simulink model "H2DFRL_LExCI_env_TD3_nosfb"  (R2023a)
settings: Solver=FixedStepAuto  StartTime=0.0  StopTime=50  FixedStep=0.08  RelTol=1e-3
values from neighbouring files (symbols this model uses):
  action_mean_selector_ppo = 1:num_actions    [ReinforcementLearningBlockInit_H2DFRL.m]
  action_sampling_mode = 1    [ReinforcementLearningBlockInit_H2DFRL.m]
  action_selector_ddpg = 1:num_actions    [ReinforcementLearningBlockInit_H2DFRL.m]
  action_std_selector_ppo = 1:num_actions    [ReinforcementLearningBlockInit_H2DFRL.m]
  action_type = 1    [ReinforcementLearningBlockInit_H2DFRL.m]
  C2C_NMPC = init_C2C_NMPC_H2DF(C2C_NMPC.expdata)    [init_H2DFRL_GRU.m]
  LowerLimit = ([0.17e-3;350;-1;1.5e-3] - C2C_NMPC.Normalization.controls.mean)./(C2C_NMPC.Normalization.controls.std)    [init_H2DFRL_GRU.m]
  num_actions = 4    [ReinforcementLearningBlockInit_H2DFRL.m]
  rl_algorithm = 2    [ReinforcementLearningBlockInit_H2DFRL.m]
  Ts = 0.08    [init_H2DFRL_GRU.m]
  UpperLimit = ([0.5e-3;900;0;5.5e-3] - C2C_NMPC.Normalization.controls.mean)./(C2C_NMPC.Normalization.controls.std)    [init_H2DFRL_GRU.m]
undefined symbols (not defined in the file or in its folder): CA50_offset, DiscIntNeverNeededParam, enable_CA50_noise, enable_CA50_offset, enable_IMEP_noise, enable_IMEP_offset, IMEP_offset, NUMBER_OF_ACTIONS
libraries: simulink x15, dspsrcs4 x4, slctrlblks x2, statsLibrary x1
(part 2 of 4)

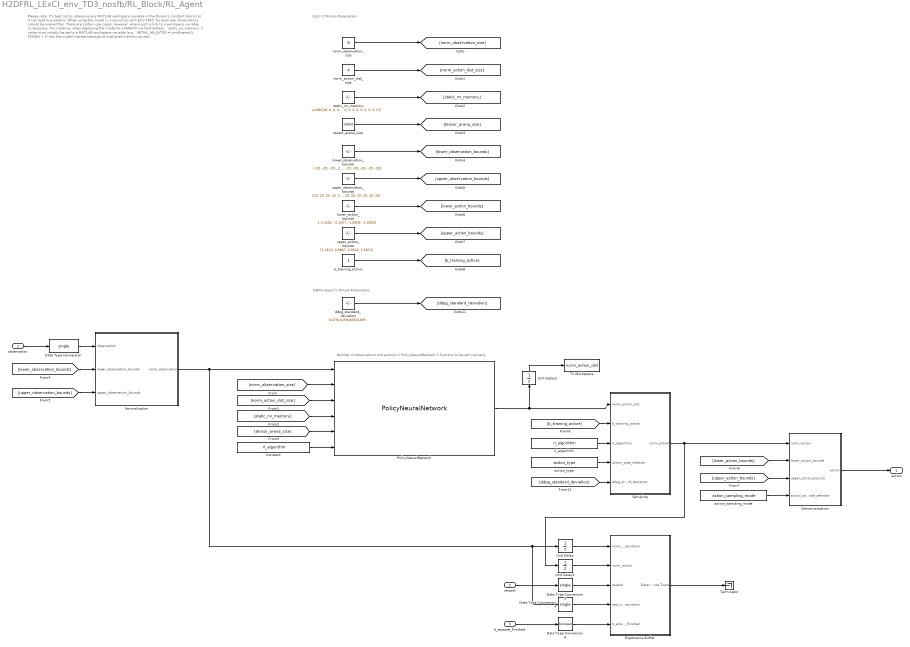
== system H2DFRL_LExCI_env_TD3_nosfb/RL_Block/RL_Agent ==
  note: LExCI 2 Minion Parameters
  note: DDPG-Specific Minion Parameters
  note: Number of observations and actions in PolicyNeuralNetwork S-Function to be set manually.
  note: Please note:
      |
      | It's best not to reference any MATLAB workspace variable in the Minion's constant blocks as it can lead to
      | problems. When using the model in conjunction with ECU-TEST, for example, those blocks cannot be
      | overwritten.
      |
      | There are certain use-cases, however, where such a link to a workspace variable is necessary. For
      | instance, when deploying the model to a MABXIII via ControlDesk, `static_nn_memory`'s value must
      | initially be set to a MATLAB workspace variable (e.g. `INITIAL_NN_BYTES = uint8(zeros(1, 65536))`). If
      | not, the model crashes because of unaligned memory access.
  observation : Inport
  reward : Inport  Port=2
  b_episode_finished : Inport  Port=3
  Constant : Constant  Value=rl_algorithm  OutDataTypeStr=uint32
  Data Type Conversion : DataTypeConversion  OutDataTypeStr=single  SaturateOnIntegerOverflow=off  RndMeth=Floor
  Data Type Conversion3 : DataTypeConversion  OutDataTypeStr=single  SaturateOnIntegerOverflow=off  RndMeth=Floor
  Data Type Conversion4 : DataTypeConversion  OutDataTypeStr=single  SaturateOnIntegerOverflow=off  RndMeth=Floor
  Data Type Conversion6 : DataTypeConversion  OutDataTypeStr=boolean  SaturateOnIntegerOverflow=off  RndMeth=Floor
  Denormalization : Subsystem
  Experience Buffer : Subsystem
  Normalization : Subsystem
  PolicyNeuralNetwork : S-Function  InitFcn=try, set_param(gcb,'FunctionName','PolicyNeuralNetwork'), end  FunctionName=PolicyNeuralNetwork  SFunctionModules=PolicyNeuralNetwork_wrapper.cpp activations activations_common add add_common add_n arg_min_max assign_variable batch_to_space_nd broadcast_args broadcast_to call_once cast ceil circular_buffer circular_buffer_common comparisons concatenation conv conv_common cumsum depth_to_space depthwise_conv depthwise_conv_common dequantize dequantize_common detection_postprocess div elementwise elu ethosu exp expand_dims fill floor floor_div floor_mod fully_connected fully_connected_common gather gather_nd hard_swish hard_swish_common if kernel_runner kernel_util_micro l2norm l2_pool_2d leaky_relu leaky_relu_common logical logical_common logistic logistic_common log_softmax lstm_eval maximum_minimum micro_tensor_utils mirror_pad mul mul_common neg pack pad pooling pooling_common prelu prelu_common quantize quantize_common read_variable reduce reduce_common reshape resize_bilinear resize_nearest_neighbor round shape slice softmax softmax_common space_to_batch_nd space_to_depth split split_v squared_difference squeeze strided_slice sub sub_common svdf svdf_common tanh transpose transpose_conv unidirectional_sequence_lstm unpack var_handle while zeros_like flatbuffer_conversions op_resolver tensor_utils error_reporter schema_utils kernel_util portable_tensor_utils quantization_util common memory_helpers all_ops_resolver micro_graph micro_error_reporter micro_context micro_profiler test_helpers recording_micro_allocator micro_interpreter micro_time micro_resource_variable test_helper_custom_ops flatbuffer_utils mock_micro_graph debug_log micro_allocation_info system_setup micro_allocator micro_string micro_utils fake_micro_context persistent_arena_buffer_allocator recording_single_arena_buffer_allocator non_persistent_arena_buffer_allocator single_arena_buffer_allocator greedy_memory_planner linear_memory_planner non_persistent_buffer_planner_shim  SFunctionDeploymentMode=off  EnableBusSupport=off  mask(S-Function Builder){}
      mask help: Simulink:masks:SFunctionBuilder_MD
      mask init:
      | val = [[.9  0.75 0.75 1 1 .9 .9 1]',[1 1 0.75 0.75 .9 .9 1 .9]'];try , sys = get_param(gcb,'SfunBuilderFcnName');if isempty(sys), sys = get_param(gcb,'FunctionName'); end,catch, sys = get_param(gcb,'FunctionName'); end
      settings: CopyFcn=set_param(gcbh,'LinkStatus','none')  PreSaveFcn=try, set_param(gcb,'FunctionName','PolicyNeuralNetwork'), end  OpenFcn=sfunctionwizard(gcbh)
      mask Display: plot(val(:,1),val(:,2)),disp(sys),port_label('input',1,'norm_observation'),port_label('input',2,'norm_observation_size'),port_label('input',3,'norm_action_dist_size'),port_label('input',4,'static_nn_memory'),port_label('input',5,'tensor_arena_size'),port_label('input',6,'rl_algorithm'),port_label('output',1,'norm_action_dist')
  Sampling : Subsystem
  Terminator : Terminator
  To Workspace : ToWorkspace  VariableName=norm_action_dist  SampleTime=-1
  Unit Delay : UnitDelay  InitialCondition=-1*ones(8,1)  SampleTime=-1  HasFrameUpgradeWarning=on
  Unit Delay1 : UnitDelay  InitialCondition=-1*ones(4,1)  SampleTime=-1  HasFrameUpgradeWarning=on
  Unit Delay2 : UnitDelay  InitialCondition=-1*ones(4,1)  SampleTime=-1  HasFrameUpgradeWarning=on
  action_sampling_mode : Constant  Value=action_sampling_mode  OutDataTypeStr=uint8
  action_type : Constant  Value=action_type  OutDataTypeStr=uint8
  b_training_active : Constant  OutDataTypeStr=boolean
  ddpg_standard_deviation : Constant  Value=0.07913259285501695  OutDataTypeStr=single
  lower_action_bounds : Constant  Value=[-2.3201, -2.1257, -1.8309, -1.6562]  OutDataTypeStr=single
  lower_observation_bounds : Constant  Value=[-20, -20, -20, -20, -20, -20, -20, -20, -20, -20, -20, -20, -20, -20, -20, -20]  OutDataTypeStr=single
  norm_action_dist_size : Constant  Value=4  OutDataTypeStr=uint32
  norm_observation_size : Constant  Value=8  OutDataTypeStr=uint32
  rl_algorithm : Constant  Value=rl_algorithm  OutDataTypeStr=uint8
  static_nn_memory : Constant  Value=uint8([28, 0, 0, 0, 84, 70, 76, 51, 0, 0, 18, 0, 28, 0, 24, 0, 20, 0, 16, 0, 12, 0, 8, 0, 0, 0, 4, 0, 18, 0, 0, 0, 24, 0, 0, 0, 104, 0, 0, 0, 140, 87, 0, 0, 156, 87, 0, 0, 228, 91, 0, 0, 3, 0, 0, 0, 2, 0, 0, 0, 44, 0, 0, 0, 4, 0, 0, 0, 40, 167, 255, 255, 12, 0, 0, 0, 4, 0, 0, 0, 19, 0, 0, 0, 67, 79, 78, 86, 69, 82, 83, 73, 79, 78, 95, 77, 69, 84, 65, 68, 65, 84, 65, 0, 76, 167, 255, 255, 11, 0, 0, 0, 4, 0, 0, 0, 19, 0, 0, 0, 109, 105, 110, 95, 114, 117, 110, 116, 105, 109, 101, 95, 118, 101, 114, 115, 105, 111, 110, 0, 13, 0, 0, 0, 32, 87, 0, 0, 0, 87, 0, 0, 232, 82, 0, 0, 216, 81, 0, 0, 200, 17, 0, 0, 184, 16, 0, 0, 168, 0, 0, 0, 160, 0, 0, 0, 152, 0, 0, 0, 144, 0, 0, 0, 136, 0, 0, 0, 104, 0, 0, 0, 4, 0, 0, 0, 54, 169, 255, 255, 4, 0, 0, 0, 84, 0, 0, 0, 12, 0, 0, 0, 8, 0, 14, 0, 8, 0, 4, 0, 8, 0, 0, 0, 16, 0, 0, 0, 36, 0, 0, 0, 0, 0, 6, 0, 8, 0, 4, 0, 6, 0, 0, 0, 4, 0, 0, 0, 0, 0, 0, 0, 0, 0, 10, 0, 16, 0, 12, 0, 8, 0, 4, 0, 10, 0, 0, 0, 2, 0, 0, 0, 2, 0, 0, 0, 4, 0, 0, 0, 6, 0, 0, 0, 50, 46, 49, 49, 46, 48, 0, 0, 150, 169, 255, 255, 4, 0, 0, 0, 16, 0, 0, 0, 49, 46, 53, 46, 48, 0, 0, 0, 0, 0, 0, 0, 0, 0, 0, 0, 80, 165, 255, 255, 84, 165, 255, 255, 88, 165, 255, 255, 92, 165, 255, 255, 194, 169, 255, 255, 4, 0, 0, 0, 0, 16, 0, 0, 161, 111, 112, 190, 191, 94, 71, 190, 9, 236, 18, 186, 150, 110, 132, 189, 195, 205, 126, 190, 160, 224, 164, 190, 220, 24, 205, 60, 91, 181, 141, 190, 4, 178, 11, 62, 5, 27, 98, 189, 159, 117, 157, 58, 80, 253, 21, 62, 26, 127, 181, 59, 190, 193, 112, 189, 3, 115, 159, 61, 17, 101, 44, 62, 224, 74, 160, 58, 205, 165, 148, 185, 158, 106, 42, 177, 126, 204, 13, 187, 114, 169, 3, 61, 244, 147, 214, 187, 184, 152, 229, 57, 110, 166, 37, 60, 191, 132, 213, 186, 230, 225, 159, 48, 97, 243, 154, 183, 115, 98, 113, 187, 183, 229, 59, 59, 20, 200, 131, 184, 169, 254, 211, 57, 155, 4, 91, 180, 39, 228, 182, 189, 148, 244, 61, 61, 219, 249, 16, 189, 166, 209, 117, 61, 248, 236, 157, 62, 218, 168, 176, 62, 136, 20, 232, 189, 26, 54, 123, 188, 4, 117, 133, 188, 177, 20, 131, 61, 163, 144, 134, 188, 252, 77, 214, 188, 38, 124, 26, 188, 41, 16, 133, 62, 22, 75, 237, 61, 232, 225, 118, 190, 58, 40, 210, 190, 116, 230, 6, 191, 172, 71, 226, 187, 191, 51, 123, 190, 128, 104, 248, 190, 129, 200, 62, 188, 242, 71, 211, 188, 65, 233, 57, 62, 196, 141, 18, 62, 252, 130, 228, 189, 154, 111, 207, 189, 147, 116, 52, 59, 242, 34, 101, 190, 67, 155, 82, 190, 235, 197, 43, 190, 107, 211, 75, 62, 128, 146, 75, 185, 217, 145, 47, 54, 248, 111, 5, 47, 180, 232, 5, 56, 127, 116, 253, 186, 182, 167, 140, 59, 46, 105, 102, 54, 155, 10, 141, 188, 136, 52, 140, 182, 235, 182, 45, 179, 232, 197, 175, 182, 175, 147, 67, 181, 58, 174, 155, 54, 37, 87, 79, 57, 218, 90, 10, 54, 14, 95, 7, 49, 142, 32, 202, 62, 194, 6, 165, 61, 172, 182, 20, 188, 166, 98, 44, 190, 83, 5, 95, 190, 240, 48, 65, 61, 151, 254, 52, 62, 53, 6, 172, 190, 148, 161, 136, 62, 129, 175, 138, 62, 159, 203, 36, 62, 251, 35, 75, 59, 196, 106, 200, 189, 174, 61, 213, 61, 28, 40, 131, 62, 172, 100, 48, 62, 176, 189, 42, 62, 213, 229, 221, 189, 46, 142, 84, 186, 254, 214, 121, 190, 5, 118, 118, 190, 245, 226, 133, 189, 0, 184, 22, 62, 80, 74, 238, 190, 250, 157, 11, 60, 191, 27, 197, 61, 111, 0, 26, 62, 246, 12, 232, 61, 119, 62, 43, 61, 254, 62, 35, 62, 117, 50, 131, 62, 11, 164, 213, 61, 100, 234, 139, 190, 67, 142, 157, 61, 150, 90, 26, 188, 236, 94, 110, 190, 4, 110, 212, 60, 183, 6, 170, 62, 40, 151, 51, 188, 3, 125, 148, 61, 103, 200, 72, 60, 166, 127, 22, 60, 28, 139, 129, 62, 46, 182, 64, 190, 18, 75, 201, 189, 224, 0, 153, 189, 238, 108, 28, 190, 62, 29, 28, 190, 93, 163, 134, 190, 229, 147, 89, 190, 70, 100, 97, 186, 40, 191, 207, 188, 112, 159, 41, 62, 187, 59, 31, 62, 224, 64, 110, 189, 91, 83, 106, 188, 221, 251, 206, 188, 117, 178, 23, 190, 91, 188, 131, 188, 14, 174, 231, 189, 112, 160, 8, 190, 140, 236, 148, 188, 191, 232, 51, 190, 133, 47, 75, 61, 243, 45, 33, 62, 143, 251, 88, 62, 97, 235, 91, 188, 82, 101, 50, 61, 128, 44, 134, 62, 238, 21, 151, 62, 138, 184, ...(+226981 chars)])  OutDataTypeStr=uint8
  tensor_arena_size : Constant  Value=100000  OutDataTypeStr=uint32
  upper_action_bounds : Constant  Value=[1.4113, 0.9867, 0.9542, 2.1874]  OutDataTypeStr=single
  upper_observation_bounds : Constant  Value=[20, 20, 20, 20, 20, 20, 20, 20, 20, 20, 20, 20, 20, 20, 20, 20]  OutDataTypeStr=single
  action : Outport
  wires:
  upper_action_bounds/1 -> [upper_action_bounds]
  PolicyNeuralNetwork/1 -> Unit Delay2/1, Sampling/1(norm_action_dist)
  upper_observation_bounds/1 -> [upper_observation_bounds]
  lower_action_bounds/1 -> [lower_action_bounds]
  [upper_observation_bounds] -> Normalization/3(upper_observation_bounds)
  [tensor_arena_size] -> PolicyNeuralNetwork/5
  b_episode_finished/1 -> Data Type Conversion6/1
  Unit Delay/1 -> Experience Buffer/1(norm_observation)
  [norm_observation_size] -> PolicyNeuralNetwork/2
  Data Type Conversion6/1 -> Experience Buffer/5(b_episode_finished)
  Unit Delay1/1 -> Experience Buffer/2(norm_action)
  Data Type Conversion3/1 -> Experience Buffer/3(reward)
  norm_observation_size/1 -> [norm_observation_size]
  Data Type Conversion/1 -> Normalization/1(observation)
  lower_observation_bounds/1 -> [lower_observation_bounds]
  Data Type Conversion4/1 -> Experience Buffer/4(new_norm_observation)
  reward/1 -> Data Type Conversion3/1
  norm_action_dist_size/1 -> [norm_action_dist_size]
  static_nn_memory/1 -> [static_nn_memory]
  Normalization/1(norm_observation) -> Unit Delay/1, Data Type Conversion4/1, PolicyNeuralNetwork/1
  observation/1 -> Data Type Conversion/1
  [norm_action_dist_size] -> PolicyNeuralNetwork/3
  [lower_observation_bounds] -> Normalization/2(lower_observation_bounds)
  tensor_arena_size/1 -> [tensor_arena_size]
  Experience Buffer/1(Experience Tuple) -> Terminator/1
  Sampling/1(norm_action) -> Unit Delay1/1, Denormalization/1(norm_action)
  Denormalization/1(action) -> action/1
  [lower_action_bounds] -> Denormalization/2(lower_action_bounds)
  [upper_action_bounds] -> Denormalization/3(upper_action_bounds)
  [static_nn_memory] -> PolicyNeuralNetwork/4
  b_training_active/1 -> [b_training_active]
  [b_training_active] -> Sampling/2(b_training_active)
  ddpg_standard_deviation/1 -> [ddpg_standard_deviation]
  action_sampling_mode/1 -> Denormalization/4(action_sampling_mode_selector)
  action_type/1 -> Sampling/4(action_type_selector)
  rl_algorithm/1 -> Sampling/3(rl_algorithm)
  [ddpg_standard_deviation] -> Sampling/5(ddpg_standard_deviation)
  Constant/1 -> PolicyNeuralNetwork/6
  Unit Delay2/1 -> To Workspace/1
